simulink model "majorChangeShift"  (R2022a)
settings: Solver=VariableStepAuto  StartTime=0.0  StopTime=18  RelTol=1e-3
PostLoadFcn:
  | postLoadCallback
InitFcn:
  | initCallback
StopFcn:
  | stopCallback
undefined symbols (not defined in the file or in its folder): modelParams
libraries: hdlsllib x7, embmathops x4, dspsrcs4 x3
CloseFcn:
  | closeCallback
settings Model: SimulationMode=accelerator  Creator=Ronnel  LastModifiedBy=Ronnel
settings DataIOCC: ReturnWorkspaceOutputs=off
settings OptimizationCC: BlockReduction=off  ConditionallyExecuteInputs=off  DefaultParameterBehavior=Inlined
settings DebuggingCC: AlgebraicLoopMsg=error
settings HardwareCC: ProdBitPerPointer=32  ProdBitPerSizeT=32  ProdBitPerPtrDiffT=32  ProdLargestAtomicFloat=None  ProdIntDivRoundTo=Undefined  ProdEndianess=Unspecified  ProdWordSize=32  ProdHWDeviceType=ASIC/FPGA->ASIC/FPGA  TargetBitPerPointer=64  TargetBitPerSizeT=64  TargetBitPerPtrDiffT=64  TargetLongLongMode=on  TargetIntDivRoundTo=Zero  TargetEndianess=LittleEndian  TargetWordSize=64  TargetHWDeviceType=Custom Processor->MATLAB Host Computer  ProdEqTarget=off

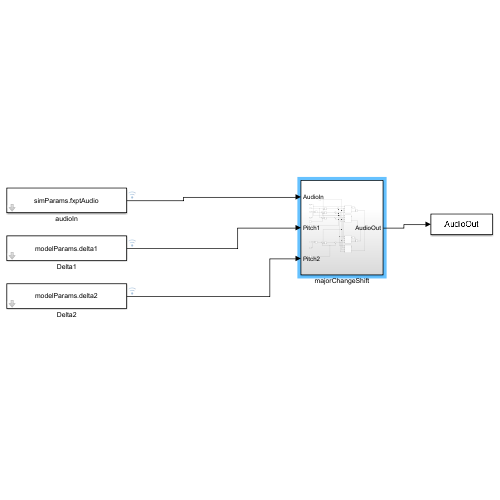
[thumbnail: Simulink's stored preview of the top-level diagram]
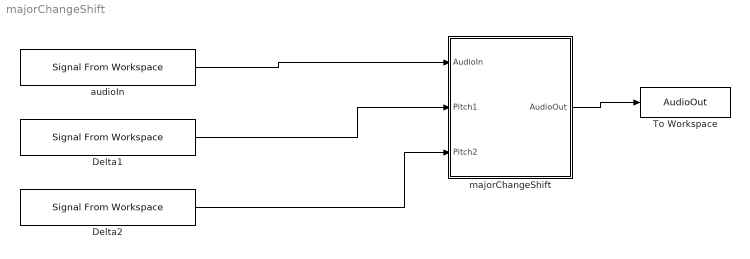
== system majorChangeShift ==
  Delta1 : dspsrcs4/Signal From Workspace  X=modelParams.delta1  Ts=modelParams.audio.samplePeriod  nsamps=1  OutputAfterFinalValue=Holding final value  ignoreOrWarnInputAndFrameLengths=off  OutputFrames=off
  Delta2 : dspsrcs4/Signal From Workspace  X=modelParams.delta2  Ts=modelParams.audio.samplePeriod  nsamps=1  OutputAfterFinalValue=Holding final value  ignoreOrWarnInputAndFrameLengths=off  OutputFrames=off
  To Workspace : ToWorkspace  VariableName=AudioOut  SampleTime=modelParams.audio.samplePeriod
      settings: Save2DSignal=2-D array (concatenate along first dimension)
  audioIn : dspsrcs4/Signal From Workspace  X=simParams.fxptAudio  Ts=modelParams.audio.samplePeriod  nsamps=1  OutputAfterFinalValue=Holding final value  ignoreOrWarnInputAndFrameLengths=off  OutputFrames=off
  majorChangeShift : Subsystem
  wires:
  audioIn/1 -> majorChangeShift/1(AudioIn)
  majorChangeShift/1(AudioOut) -> To Workspace/1
  Delta1/1 -> majorChangeShift/2(Pitch1)
  Delta2/1 -> majorChangeShift/3(Pitch2)

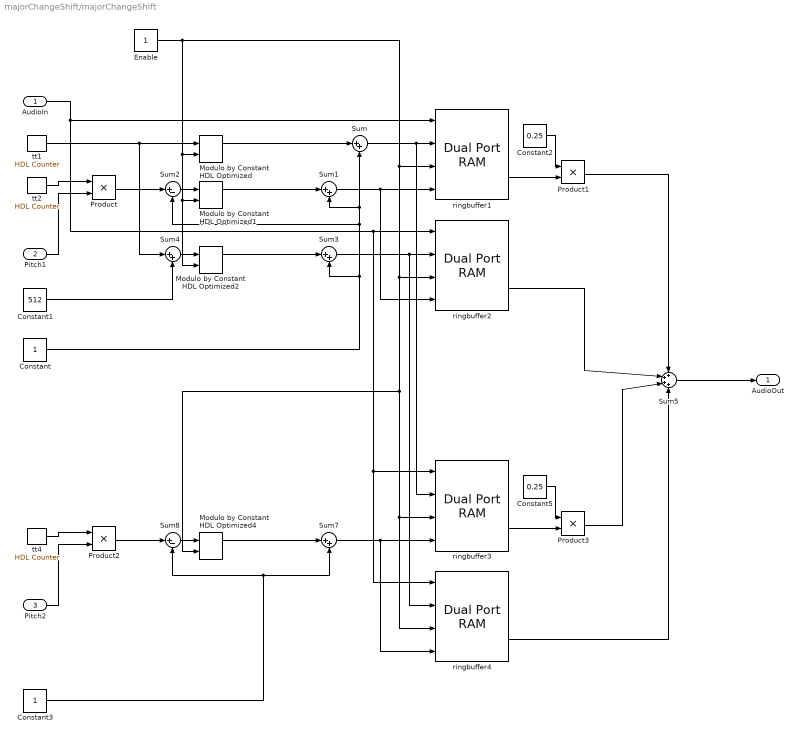
== system majorChangeShift/majorChangeShift ==
  AudioIn : Inport  SampleTime=modelParams.audio.samplePeriod
  Pitch1 : Inport  Port=2  SampleTime=modelParams.audio.samplePeriod
  Pitch2 : Inport  Port=3  SampleTime=modelParams.audio.samplePeriod
  Constant : Constant  OutDataTypeStr=uint32  SampleTime=modelParams.audio.samplePeriod
  Constant1 : Constant  Value=512  OutDataTypeStr=uint32  SampleTime=modelParams.audio.samplePeriod
  Constant2 : Constant  Value=0.25  OutDataTypeStr=fixdt(0,modelParams.audio.wordLength,modelParams.audio.fractionLength)  SampleTime=modelParams.audio.samplePeriod
  Constant3 : Constant  OutDataTypeStr=uint32  SampleTime=modelParams.audio.samplePeriod
  Constant5 : Constant  Value=0.25  OutDataTypeStr=fixdt(0,modelParams.audio.wordLength,modelParams.audio.fractionLength)  SampleTime=modelParams.audio.samplePeriod
  Enable : Constant  OutDataTypeStr=boolean  SampleTime=modelParams.audio.samplePeriod
  Modulo by Constant HDL Optimized{,1..2,4} (4 alike) : embmathops/Modulo by Constant HDL Optimized  Denominator=modelParams.buffer_size  SimulateUsing=Code generation
      settings: SourceProductBaseCode=SL
  Product : Product  SampleTime=modelParams.audio.samplePeriod
  Product1 : Product  OutDataTypeStr=fixdt(1,modelParams.audio.wordLength,modelParams.audio.fractionLength)  SaturateOnIntegerOverflow=on  SampleTime=modelParams.audio.samplePeriod
  Product2 : Product  SampleTime=modelParams.audio.samplePeriod
  Product3 : Product  OutDataTypeStr=fixdt(1,modelParams.audio.wordLength,modelParams.audio.fractionLength)  SaturateOnIntegerOverflow=on  SampleTime=modelParams.audio.samplePeriod
  Sum{,1,3..4,7} (5 alike) : Sum  Inputs=|++  OutDataTypeStr=fixdt(0,modelParams.dpramAddressSize,0)  SampleTime=modelParams.audio.samplePeriod
  Sum2 : Sum  Inputs=|+-  OutDataTypeStr=fixdt(0,modelParams.dpramAddressSize,0)  SampleTime=modelParams.audio.samplePeriod
  Sum5 : Sum  Inputs=++++  OutDataTypeStr=fixdt(1,modelParams.audio.wordLength,modelParams.audio.fractionLength)  SaturateOnIntegerOverflow=on  SampleTime=modelParams.audio.samplePeriod
  Sum8 : Sum  Inputs=|+-  OutDataTypeStr=fixdt(0,modelParams.dpramAddressSize,0)  SampleTime=modelParams.audio.samplePeriod
  ringbuffer{1..4} (4 alike) : hdlsllib/HDL RAMs/Dual Port RAM  ram_size=modelParams.dpramAddressSize
      settings: SourceProductBaseCode=SL
  tt1 : hdlsllib/Sources/HDL Counter  CountType=Free running  CountInit=1  CountStep=1  CountMax=25  CountFromType=Initial value  CountFrom=1  CountResetPort=off  CountLoadPort=off  CountEnbPort=off  CountDirPort=off  CountHitOutputPort=off  CountDataType=Unsigned  CountWordLen=modelParams.dpramAddressSize  CountFracLen=0  CountSampTime=modelParams.audio.samplePeriod
  tt2 : hdlsllib/Sources/HDL Counter  CountType=Free running  CountInit=1  CountStep=1  CountMax=25  CountFromType=Initial value  CountFrom=1  CountResetPort=off  CountLoadPort=off  CountEnbPort=off  CountDirPort=off  CountHitOutputPort=off  CountDataType=Unsigned  CountWordLen=32  CountFracLen=0  CountSampTime=modelParams.audio.samplePeriod
  tt4 : hdlsllib/Sources/HDL Counter  CountType=Free running  CountInit=1  CountStep=1  CountMax=25  CountFromType=Initial value  CountFrom=1  CountResetPort=off  CountLoadPort=off  CountEnbPort=off  CountDirPort=off  CountHitOutputPort=off  CountDataType=Unsigned  CountWordLen=32  CountFracLen=0  CountSampTime=modelParams.audio.samplePeriod
  AudioOut : Outport  SampleTime=modelParams.audio.samplePeriod
  wires:
  AudioIn/1 -> ringbuffer1/1, ringbuffer4/1, ringbuffer3/1, ringbuffer2/1
  tt1/1 -> Sum4/1, Modulo by Constant HDL Optimized/1
  Constant/1 -> Sum3/2, Sum2/2, Sum1/2, Sum/2
  Modulo by Constant HDL Optimized/1 -> Sum/1
  Sum1/1 -> ringbuffer1/4, ringbuffer2/4
  Modulo by Constant HDL Optimized1/1 -> Sum1/1
  Sum2/1 -> Modulo by Constant HDL Optimized1/1
  tt2/1 -> Product/1
  Pitch1/1 -> Product/2
  Product/1 -> Sum2/1
  Sum3/1 -> ringbuffer2/2, ringbuffer4/2
  Modulo by Constant HDL Optimized2/1 -> Sum3/1
  Sum4/1 -> Modulo by Constant HDL Optimized2/1
  Constant1/1 -> Sum4/2
  Constant2/1 -> Product1/1
  Product1/1 -> Sum5/1
  Sum5/1 -> AudioOut/1
  ringbuffer1/2 -> Product1/2
  ringbuffer2/2 -> Sum5/2
  ringbuffer4/2 -> Sum5/4
  ringbuffer3/2 -> Product3/2
  Pitch2/1 -> Product2/2
  Product3/1 -> Sum5/3
  Constant5/1 -> Product3/1
  Sum7/1 -> ringbuffer3/4, ringbuffer4/4
  Sum/1 -> ringbuffer3/2, ringbuffer1/2
  tt4/1 -> Product2/1
  Sum8/1 -> Modulo by Constant HDL Optimized4/1
  Product2/1 -> Sum8/1
  Modulo by Constant HDL Optimized4/1 -> Sum7/1
  Enable/1 -> Modulo by Constant HDL Optimized2/2, Modulo by Constant HDL Optimized1/2, Modulo by Constant HDL Optimized/2, ringbuffer1/3, ringbuffer2/3, Modulo by Constant HDL Optimized4/2, ringbuffer3/3, ringbuffer4/3
  Constant3/1 -> Sum7/2, Sum8/2
